simulink model "exam"  (R2022b)
settings: Solver=VariableStepAuto  StartTime=0.0  StopTime=10.0  RelTol=1e-3
settings Model: Creator=devak  LastModifiedBy=devak

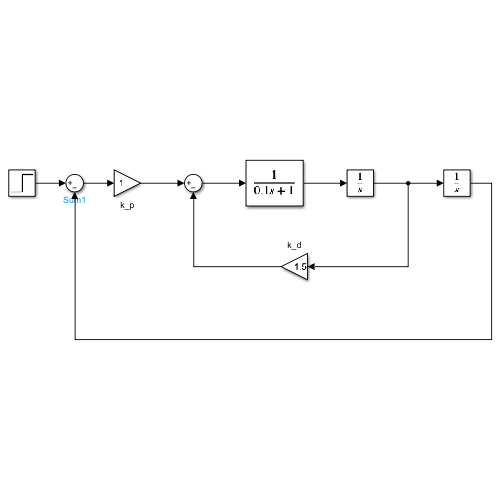
[thumbnail: Simulink's stored preview of the top-level diagram]
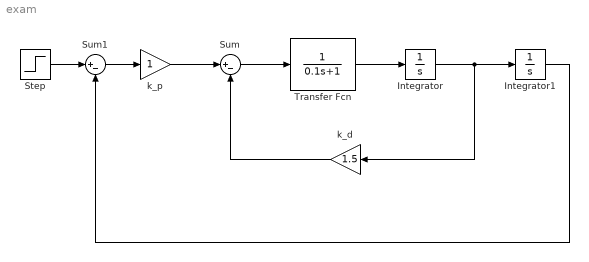
== system exam ==
  Integrator : Integrator
  Integrator1 : Integrator
  Step : Step  SampleTime=0
  Sum : Sum  Inputs=|+-
  Sum1 : Sum  Inputs=|+-
  Transfer Fcn : TransferFcn  Denominator=[0.1 1]
  k_d : Gain  Gain=1.5
  k_p : Gain
  wires:
  k_p/1 -> Sum/1
  k_d/1 -> Sum/2
  Integrator/1 -> k_d/1, Integrator1/1
  Transfer Fcn/1 -> Integrator/1
  Sum/1 -> Transfer Fcn/1
  Step/1 -> Sum1/1
  Integrator1/1 -> Sum1/2
  Sum1/1 -> k_p/1
